simulink model "untitled"  (R2014a)
settings: Solver=ode45  StartTime=0.0  StopTime=30  MaxStep=0.001  MinStep=0.0001  RelTol=1e-3
settings Model: Creator=Valentin  LastModifiedBy=Valentin

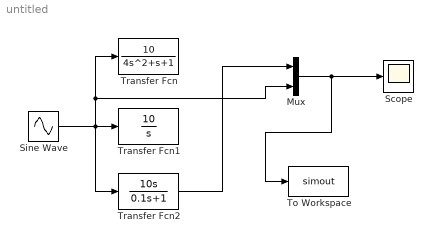
== system untitled ==
  Mux : Mux  Inputs=2
  Scope : Scope
  Sine Wave : Sin  Frequency=2  SampleTime=0
  To Workspace : ToWorkspace  VariableName=simout  SaveFormat=Timeseries  SampleTime=-1
  Transfer Fcn : TransferFcn  Numerator=[10]  Denominator=[4 1 1]
  Transfer Fcn1 : TransferFcn  Numerator=[10]  Denominator=[1 0]
  Transfer Fcn2 : TransferFcn  Numerator=[10 0]  Denominator=[0.1 1]
  wires:
  Sine Wave/1 -> Transfer Fcn2/1, Transfer Fcn/1, Mux/2, Transfer Fcn1/1
  Mux/1 -> To Workspace/1, Scope/1
  Transfer Fcn2/1 -> Mux/1
